simulink model "cargaRLC_variable"  (R2018a)
settings: Solver=ode4  StartTime=0.0  StopTime=10.0  FixedStep=1e-4  RelTol=1e-3
libraries: simulink x2, powerlib_meascontrol x1
settings Model: Creator=MarioAndres  LastModifiedBy=cmparedes
settings OptimizationCC: DefaultParameterBehavior=Inlined  EnhancedBackFolding=on  PassReuseOutputArgsAs=Individual arguments  OptimizeBlockOrder=speed  DifferentSizesBufferReuse=on  OptimizationCustomize=off
settings DebuggingCC: ParameterTunabilityLossMsg=error
settings SFSimCC: MATLABDynamicMemAlloc=off
settings RTWCC: SystemTargetFile=ert.tlc  TemplateMakefile=ert_default_tmf  GenerateReport=on  IncludeHyperlinkInReport=on  LaunchReport=on  GenerateTraceInfo=on  GenerateTraceReport=on  GenerateTraceReportSl=on  GenerateTraceReportSf=on  GenerateTraceReportEml=on
settings CodeAppCC: ForceParamTrailComments=on  IgnoreCustomStorageClasses=off  OperatorAnnotations=on  SimulinkDataObjDesc=on  SFDataObjDesc=on  InsertBlockDesc=on
settings ERTTargetCC: TargetLangStandard=C99 (ISO)  GenerateSampleERTMain=on  SupportContinuousTime=on  InlinedParameterPlacement=NonHierarchical  ERTCustomFileTemplate=example_file_process.tlc

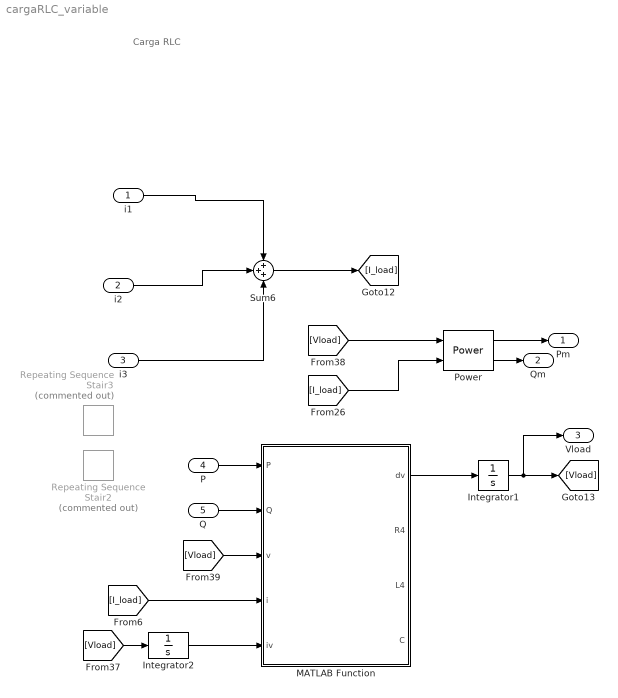
== system cargaRLC_variable ==
  note: Carga RLC
  i1 : Inport
  i2 : Inport  Port=2
  i3 : Inport  Port=3
  P : Inport  Port=4
  Q : Inport  Port=5
  Integrator1 : Integrator  UpperSaturationLimit=400  LowerSaturationLimit=-400
  Integrator2 : Integrator
  MATLAB Function : MATLAB Function  TreatAsAtomicUnit=on
  Power : powerlib_meascontrol/Measurements/Power  Freq=60  Vinit=[1, 0]  Iinit=[1, 0]  Ts=0
      settings: SourceProductName=Simscape Power Systems
  Repeating Sequence Stair2 : simulink/Sources/Repeating Sequence Stair  Commented=on  OutValues=[-4000 -2000 -7000 -6000 -5000 -4000 -3000 -2000].'  tsamp=10  OutMin=[]  OutMax=[]  OutDataTypeStr=double  OutputDataTypeScalingMode=double  OutDataType=fixdt(0,8)  ConRadixGroup=Best Precision: Vector-wise  OutScaling=2^-12
  Repeating Sequence Stair3 : simulink/Sources/Repeating Sequence Stair  Commented=on  OutValues=[1000 2000 3000 4000 5000 6000 7000 8000].'  tsamp=10  OutMin=[]  OutMax=[]  OutDataTypeStr=double  OutputDataTypeScalingMode=double  OutDataType=fixdt(0,8)  ConRadixGroup=Best Precision: Vector-wise  OutScaling=2^-12
  Sum6 : Sum  Inputs=3
  Pm : Outport
  Qm : Outport  Port=2
  Vload : Outport  Port=3
  wires:
  [I_load] -> MATLAB Function/4(i)
  [Vload] -> Integrator2/1
  [Vload] -> MATLAB Function/3(v)
  Integrator2/1 -> MATLAB Function/5(iv)
  [Vload] -> Power/1
  MATLAB Function/1(dv) -> Integrator1/1
  [I_load] -> Power/2
  i1/1 -> Sum6/1
  i3/1 -> Sum6/3
  Sum6/1 -> [I_load]
  Integrator1/1 -> Vload/1, [Vload]
  i2/1 -> Sum6/2
  Power/2 -> Qm/1
  Power/1 -> Pm/1
  P/1 -> MATLAB Function/1(P)
  Q/1 -> MATLAB Function/2(Q)

== matlab function cargaRLC_variable/MATLAB Function ==
  data: P input; dv output; Q input; v input; i input; iv input; R4 output; L4 output; C output
function [dv,R4,L4,C]= fcn(P,Q,v,i,iv)
Vrms=170/sqrt(2);
w=2*pi*60;

% R1=Vrms^2/(0.7*P);
R1=Vrms^2/P;
R2=Vrms^2/(0.3*P);
% R3=Vrms^2/(0.99*P);
if Q>=0
    R3=5;
    L=Vrms^2/(w*1.3*Q);
    %L=Vrms^2/(w*Q);
    C=0.3*Q/(w*Vrms^2);
else
    R3=-1;
    L=Vrms^2/(w*0.3*abs(Q));
    C=1.3*abs(Q)/(w*Vrms^2);
end
R4=R1;
L4=L;

dv=(R4*L4*i-L4*v-R4*iv)/(R4*L4*C);
